simulink model "CSTR_gen_UA_err"  (R2020a)
settings: Solver=VariableStepAuto  StartTime=0.0  StopTime=dur  RelTol=1e-3
values from neighbouring files (symbols this model uses):
  Ca_i = 1    [CSTR_In.mat]
  CaSwitch = 0    [CSTR_Data_Generation.m]    (also in CSTR_Data_loops_UA_err.m)
  EaR = 8750    [CSTR_In.mat]
  H = 50000    [CSTR_In.mat]
  HA = 50000    [CSTR_In.mat]
  HD = 239    [CSTR_In.mat]
  k0Switch = 0    [CSTR_Data_Generation.m]    (also in CSTR_Data_loops_UA_err.m)
  k_0 = 72000000000    [CSTR_In.mat]
  serr = 0    [CSTR_Data_Generation.m]    (also in CSTR_Data_loops_UA_err.m)
  t_samp = 1    [CSTR_Data_Generation.m]    (also in CSTR_Data_loops_UA_err.m)
  t_Tj = 0    [CSTR_Data_Generation.m]    (also in CSTR_Data_loops_UA_err.m)
  Tj_i = 290    [CSTR_Data_Generation.m]    (also in CSTR_Data_loops_UA_err.m)
  Tj_o = Tj_i    (= 290)    [CSTR_Data_Generation.m]    (also in CSTR_Data_loops_UA_err.m)
  UASwitch = 1    [CSTR_Data_Generation.m]    (also in CSTR_Data_loops_UA_err.m)
  V = 100    [CSTR_In.mat]
libraries: simulink x7
settings Model: Creator=20029586  LastModifiedBy=20029586
settings DataIOCC: ReturnWorkspaceOutputs=off
settings DebuggingCC: ArithmeticOperatorsInVariantConditions=warning
settings SFSimCC: CustomCodeUndefinedFunction=UseInterfaceOnly
settings CodeAppCC: StateflowObjectComments=on

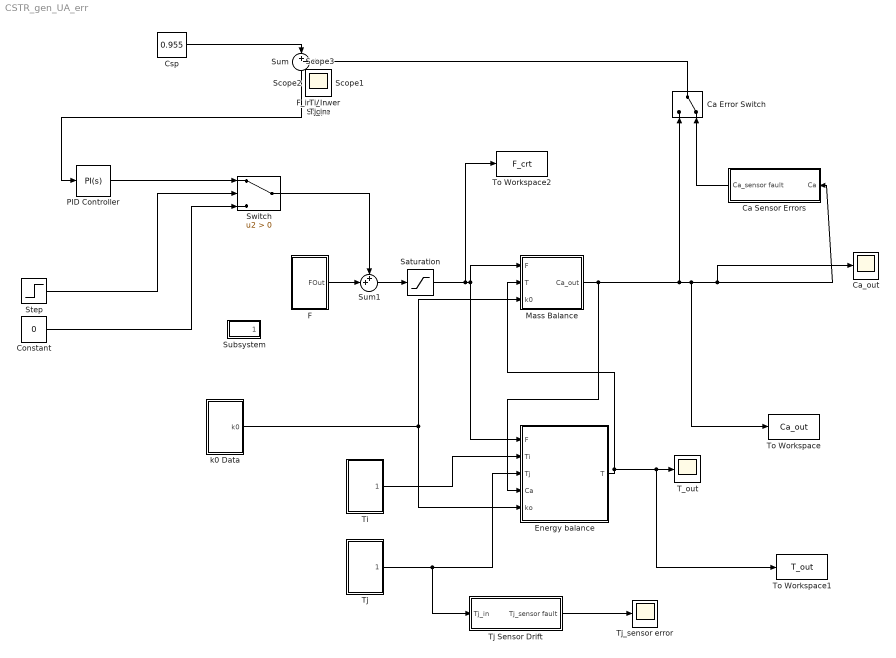
== system CSTR_gen_UA_err ==
  Ca Error Switch : ManualSwitch  CurrentSetting=0
  Ca Sensor Errors : Subsystem
  Ca_out : Scope
  Constant : Constant  Value=0
  Csp : Constant  Value=0.955
  Energy balance : Subsystem
  F : Subsystem
  Mass Balance : Subsystem
  PID Controller : simulink/Continuous/PID Controller  Controller=PI  Form=Parallel  TimeDomain=Continuous-time  UseExternalTs=off  SampleTime=-1  IntegratorMethod=Forward Euler  FilterMethod=Forward Euler  ControllerParametersSource=internal  P=5  I=50  D=0  UseFilter=on  N=100  TunerSelectOption=Transfer Function Based (PID Tuner App)  InitialConditionSource=internal  InitialConditionForIntegrator=0  InitialConditionForFilter=0  DifferentiatorICPrevScaledInput=0  ExternalReset=none  TrackingMode=off  Kt=1  LimitOutput=off  UpperSaturationLimit=inf  LowerSaturationLimit=-inf  LinearizeAsGain=on  AntiWindupMode=none  Kb=1  POutMin=[]  POutMax=[]  IOutMin=[]  IOutMax=[]  DOutMin=[]  DOutMax=[]  NOutMin=[]  NOutMax=[]  SumOutMin=[]  SumOutMax=[]  SaturationOutMin=[]  SaturationOutMax=[]  PParamMin=[]  PParamMax=[]  IParamMin=[]  IParamMax=[]  DParamMin=[]  DParamMax=[]  NParamMin=[]  NParamMax=[]  KbParamMin=[]  KbParamMax=[]  KtParamMin=[]  KtParamMax=[]  KbOutMin=[]  KbOutMax=[]  KtOutMin=[]  KtOutMax=[]  IntegratorOutMin=[]  IntegratorOutMax=[]  FilterOutMin=[]  FilterOutMax=[]  SumI1OutMin=[]  SumI1OutMax=[]  SumI2OutMin=[]  SumI2OutMax=[]  SumI3OutMin=[]  SumI3OutMax=[]  SumI4OutMin=[]  SumI4OutMax=[]  SumDOutMin=[]  SumDOutMax=[]  DifferentiatorOutMin=[]  DifferentiatorOutMax=[]  FilterDiffOutCoefMin=[]  FilterDiffOutCoefMax=[]  ReciprocalOutMin=[]  ReciprocalOutMax=[]  SumDenOutMin=[]  SumDenOutMax=[]  SumNumOutMin=[]  SumNumOutMax=[]  DivideOutMin=[]  DivideOutMax=[]  UdiffTsProdOutMin=[]  UdiffTsProdOutMax=[]  NTsProdOutMin=[]  NTsProdOutMax=[]  UintegralTsProdOutMin=[]  UintegralTsProdOutMax=[]  UngainTsProdOutMin=[]  UngainTsProdOutMax=[]  IntegratorContinuousStateAttributes=''  IntegratorStateMustResolveToSignalObject=off  IntegratorRTWStateStorageClass=Auto  FilterContinuousStateAttributes=''  FilterStateMustResolveToSignalObject=off  FilterRTWStateStorageClass=Auto  ParallelPVariant=InternalParameters  IdealPVariant=Disabled  IVariant=InternalParameters  DVariant=Disabled  IntegratorVariant=Continuous  SatVariant=Disabled  AWVariant=Passthrough  PCopyVariant=Disabled  TRVariant=Disabled  FdbkBlocksVariant=Forward  IdealPFdbkVariant=Disabled  SatFdbkVariant=Disabled  DerivativeFilterVariant=Disabled  NVariant=Disabled  NCopyVariant=Disabled_SignalSpec  FilterICVariant=Disabled  IntegratorICVariant=InternalICs  ExternalResetVariant=Disabled  TRSumVariant=Passthrough  SumFdbkVariant=Disabled  SumVariant=Sum_PI  TsampFilterVariant=InternalTs  TsampNgainVariant=Passthrough  TsampIntegralVariant=Passthrough
  Saturation : Saturate  UpperLimit=5000  LowerLimit=0
  Step : Step  Time=0  Before=-1  SampleTime=0
  Subsystem : Subsystem
  Sum : Sum  Inputs=|+-
  Sum1 : Sum  Inputs=++|
  Switch : Switch  Criteria=u2 > Threshold
  T_out : Scope
  Ti : Subsystem
  Tj : Subsystem
  Tj Sensor Drift : Subsystem
  Tj_sensor error : Scope
  To Workspace : ToWorkspace  VariableName=Ca_out  SaveFormat=Timeseries  SampleTime=t_samp
  To Workspace1 : ToWorkspace  VariableName=T_out  SaveFormat=Timeseries  SampleTime=t_samp
  To Workspace2 : ToWorkspace  VariableName=F_crt  SaveFormat=Timeseries  SampleTime=t_samp
  k0 Data : Subsystem
  F_in Viewer : Scope
  Scope{,1..3} (4 alike) : Scope
  Ti_In : Scope
  Tj_in : Scope
  wires:
  Energy balance/1(T) -> To Workspace1/1, T_out/1, Mass Balance/2(T)
  Ti/1(Ti_Out) -> Energy balance/2(Ti)
  Tj/1(Tj_Out) -> Tj Sensor Drift/1(Tj_in), Energy balance/3(Tj)
  Mass Balance/1(Ca_out) -> Ca Sensor Errors/1(Ca), Ca_out/1, To Workspace/1, Ca Error Switch/1, Energy balance/4(Ca)
  Csp/1 -> Sum/1
  F/1(FOut) -> Sum1/2
  Tj Sensor Drift/1(Tj_sensor fault) -> Tj_sensor error/1
  Ca Error Switch/1 -> Sum/2
  Ca Sensor Errors/1(Ca_sensor fault) -> Ca Error Switch/2
  Switch/1 -> Sum1/1
  Constant/1 -> Switch/3
  Step/1 -> Switch/2
  Saturation/1 -> Energy balance/1(F), Mass Balance/1(F), To Workspace2/1
  Sum1/1 -> Saturation/1
  k0 Data/1(k0) -> Mass Balance/3(k0), Energy balance/5(ko)
  PID Controller/1 -> Switch/1
  Sum/1 -> PID Controller/1

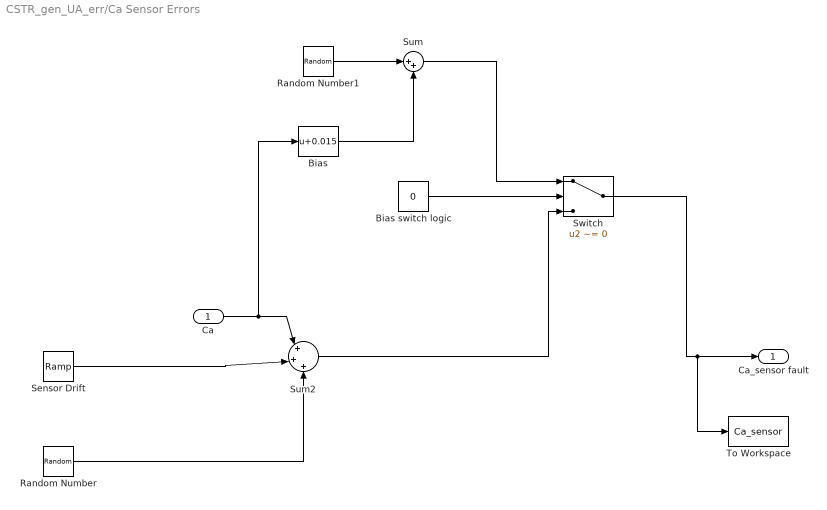
== system CSTR_gen_UA_err/Ca Sensor Errors ==
  Ca : Inport
  Bias : Bias  Bias=0.015
  Bias switch logic : Constant  Value=0
  Random Number : RandomNumber  Variance=0.0001  SampleTime=0.1
  Random Number1 : RandomNumber  Variance=1*10^-6  SampleTime=0.1
  Sensor Drift : simulink/Sources/Ramp  slope=serr  start=t_serr  InitialOutput=0
  Sum : Sum  Inputs=|++
  Sum2 : Sum  Inputs=|+|+|+
  Switch : Switch  Criteria=u2 ~= 0
  To Workspace : ToWorkspace  VariableName=Ca_sensor  SaveFormat=Timeseries  SampleTime=t_samp
  Ca_sensor fault : Outport
  wires:
  Ca/1 -> Bias/1, Sum2/1
  Sensor Drift/1 -> Sum2/2
  Sum2/1 -> Switch/3
  Random Number/1 -> Sum2/3
  Random Number1/1 -> Sum/1
  Bias/1 -> Sum/2
  Sum/1 -> Switch/1
  Bias switch logic/1 -> Switch/2
  Switch/1 -> To Workspace/1, Ca_sensor fault/1

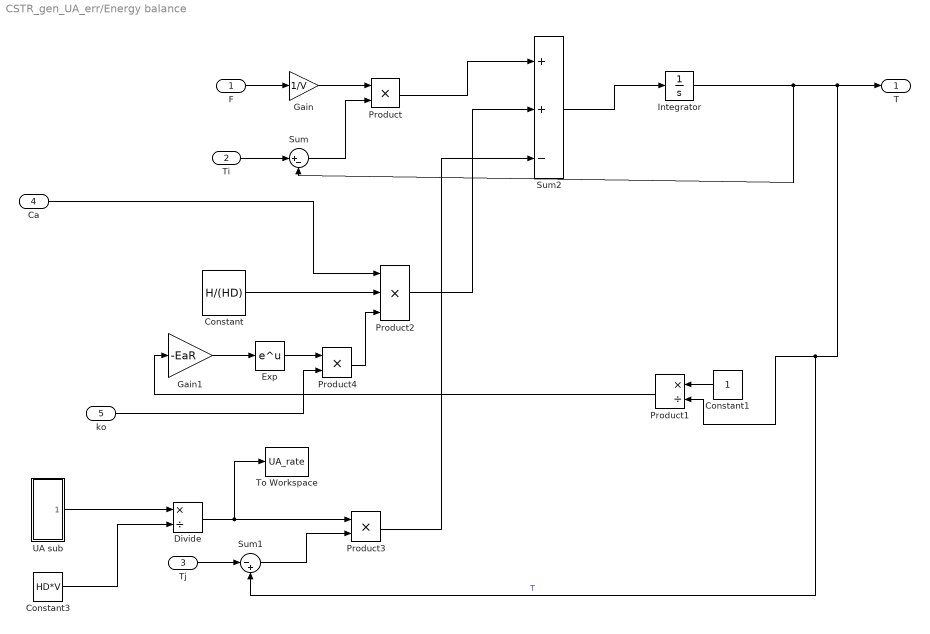
== system CSTR_gen_UA_err/Energy balance ==
  F : Inport
  Ti : Inport  Port=2
  Tj : Inport  Port=3
  Ca : Inport  Port=4
  ko : Inport  Port=5
  Constant : Constant  Value=H/(HD)
  Constant1 : Constant
  Constant3 : Constant  Value=HD*V
  Divide : Product  Inputs=*/
  Exp : Math  SignedPower=on  SaturateOnIntegerOverflow=on
  Gain : Gain  Gain=1/V
  Gain1 : Gain  Gain=-EaR
  Integrator : Integrator  InitialCondition=312.4
  Product : Product
  Product1 : Product  Inputs=*/
  Product2 : Product  Inputs=3
  Product3 : Product
  Product4 : Product
  Sum : Sum  Inputs=|+-
  Sum1 : Sum  Inputs=|-+
  Sum2 : Sum  Inputs=|++-
  To Workspace : ToWorkspace  VariableName=UA_rate  SaveFormat=Timeseries  SampleTime=t_samp
  UA sub : Subsystem
  T : Outport
  wires:
  Integrator/1 -> Sum/2, Sum1/2, Product1/2, T/1  "T"
  F/1 -> Gain/1
  Gain/1 -> Product/1
  Ti/1 -> Sum/1
  Sum/1 -> Product/2
  Constant1/1 -> Product1/1
  Product1/1 -> Gain1/1
  Gain1/1 -> Exp/1
  Exp/1 -> Product4/1
  Constant/1 -> Product2/2
  Product4/1 -> Product2/3
  Divide/1 -> To Workspace/1, Product3/1
  Tj/1 -> Sum1/1
  Sum1/1 -> Product3/2
  Product/1 -> Sum2/1
  Product2/1 -> Sum2/2
  Product3/1 -> Sum2/3
  Sum2/1 -> Integrator/1
  Ca/1 -> Product2/1
  ko/1 -> Product4/2
  Constant3/1 -> Divide/2
  UA sub/1(Out1) -> Divide/1

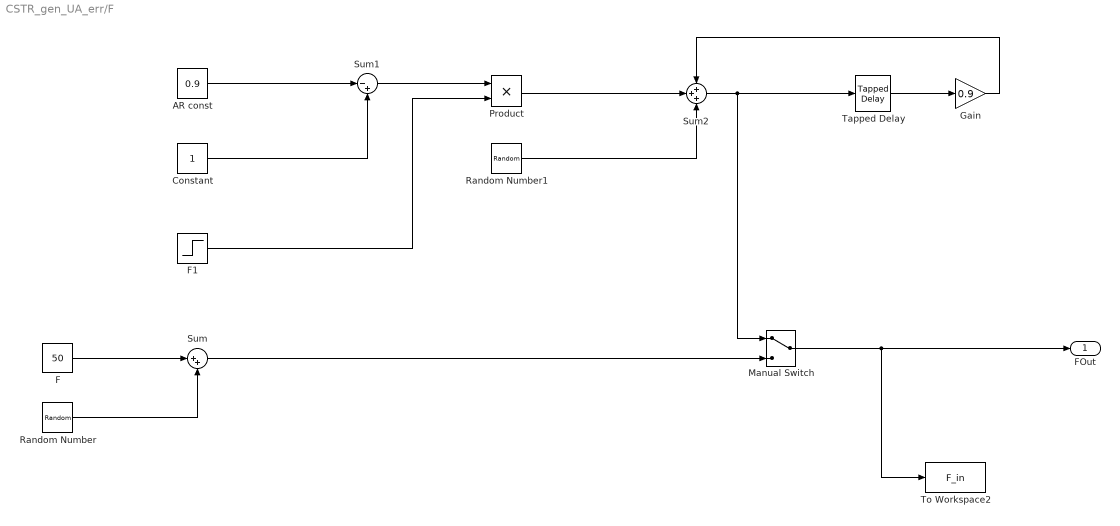
== system CSTR_gen_UA_err/F ==
  AR const : Constant  Value=0.9
  Constant : Constant
  F : Constant  Value=50
  F1 : Step  Time=0  Before=50  After=50  SampleTime=0
  Gain : Gain  Gain=0.9
  Manual Switch : ManualSwitch
  Product : Product
  Random Number : RandomNumber  Variance=1.9  SampleTime=0.1
  Random Number1 : RandomNumber  Variance=1.9  SampleTime=0.1
  Sum : Sum  Inputs=|++
  Sum1 : Sum  Inputs=|-+
  Sum2 : Sum  Inputs=+++
  Tapped Delay : simulink/Discrete/Tapped Delay  vinit=50  samptime=0.1  NumDelays=1  DelayOrder=Oldest  includeCurrent=off
  To Workspace2 : ToWorkspace  VariableName=F_in  SaveFormat=Timeseries  SampleTime=t_samp
  FOut : Outport
  wires:
  F/1 -> Sum/1
  Sum/1 -> Manual Switch/2
  Manual Switch/1 -> To Workspace2/1, FOut/1
  Random Number/1 -> Sum/2
  AR const/1 -> Sum1/1
  Constant/1 -> Sum1/2
  Sum1/1 -> Product/1
  F1/1 -> Product/2
  Product/1 -> Sum2/2
  Random Number1/1 -> Sum2/3
  Sum2/1 -> Manual Switch/1, Tapped Delay/1
  Tapped Delay/1 -> Gain/1
  Gain/1 -> Sum2/1

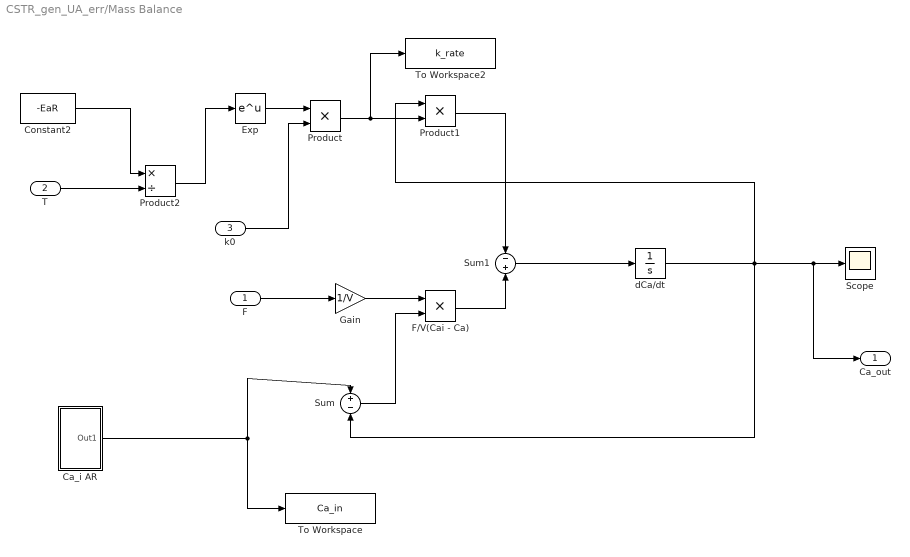
== system CSTR_gen_UA_err/Mass Balance ==
  F : Inport
  T : Inport  Port=2
  k0 : Inport  Port=3
  Ca_i AR : Subsystem
  Constant2 : Constant  Value=-EaR
  Exp : Math  SignedPower=on  SaturateOnIntegerOverflow=on
  F/V(Cai - Ca) : Product
  Gain : Gain  Gain=1/V
  Product : Product
  Product1 : Product
  Product2 : Product  Inputs=*/
  Scope : Scope
  Sum : Sum  Inputs=+-
  Sum1 : Sum  Inputs=-+
  To Workspace : ToWorkspace  VariableName=Ca_in  SaveFormat=Timeseries  SampleTime=t_samp
  To Workspace2 : ToWorkspace  VariableName=k_rate  SaveFormat=Timeseries  SampleTime=t_samp
  dCa/dt : Integrator  InitialCondition=0.952
  Ca_out : Outport
  wires:
  Product/1 -> To Workspace2/1, Product1/2
  Product1/1 -> Sum1/1
  Sum/1 -> F/V(Cai - Ca)/2
  dCa/dt/1 -> Ca_out/1, Scope/1, Sum/2, Product1/1
  Gain/1 -> F/V(Cai - Ca)/1
  Sum1/1 -> dCa/dt/1
  F/1 -> Gain/1
  Exp/1 -> Product/1
  F/V(Cai - Ca)/1 -> Sum1/2
  Constant2/1 -> Product2/1
  Product2/1 -> Exp/1
  T/1 -> Product2/2
  Ca_i AR/1(Out1) -> Sum/1, To Workspace/1
  k0/1 -> Product/2

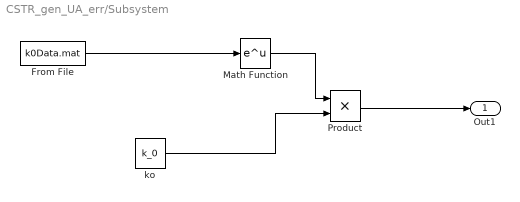
== system CSTR_gen_UA_err/Subsystem ==
  From File : FromFile  FileName=k0Data.mat  SampleTime=0.01
  Math Function : Math  SignedPower=on  SaturateOnIntegerOverflow=on
  Product : Product
  ko : Constant  Value=k_0
  Out1 : Outport
  wires:
  Math Function/1 -> Product/1
  Product/1 -> Out1/1
  From File/1 -> Math Function/1
  ko/1 -> Product/2

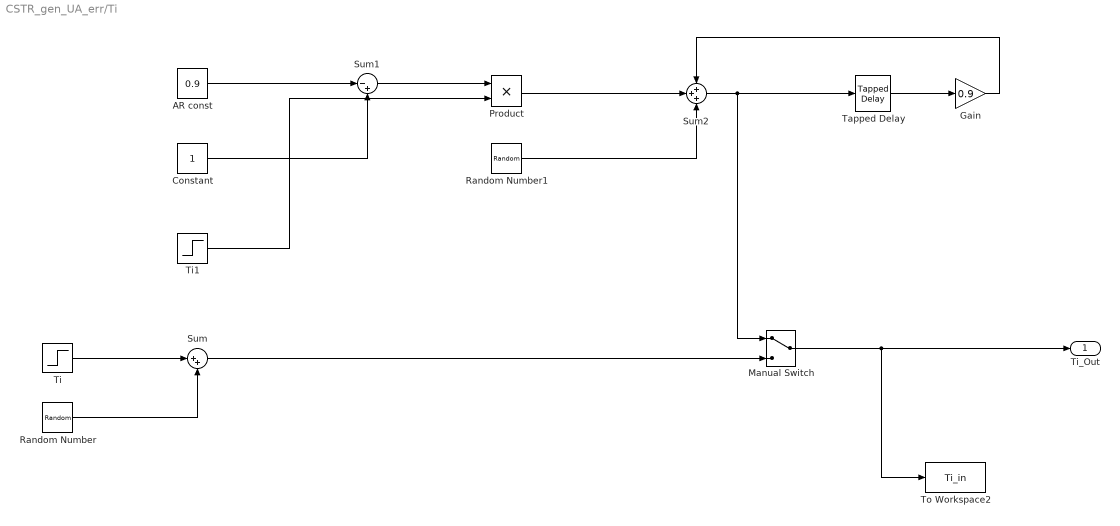
== system CSTR_gen_UA_err/Ti ==
  AR const : Constant  Value=0.9
  Constant : Constant
  Gain : Gain  Gain=0.9
  Manual Switch : ManualSwitch
  Product : Product
  Random Number : RandomNumber  Variance=0.475  SampleTime=0.1
  Random Number1 : RandomNumber  Variance=0.475  SampleTime=0.1
  Sum : Sum  Inputs=|++
  Sum1 : Sum  Inputs=|-+
  Sum2 : Sum  Inputs=+++
  Tapped Delay : simulink/Discrete/Tapped Delay  vinit=350  samptime=0.1  NumDelays=1  DelayOrder=Oldest  includeCurrent=off
  Ti : Step  Time=0  Before=350  After=350  SampleTime=0
  Ti1 : Step  Time=0  Before=350  After=350  SampleTime=0
  To Workspace2 : ToWorkspace  VariableName=Ti_in  SaveFormat=Timeseries  SampleTime=t_samp
  Ti_Out : Outport
  wires:
  Ti/1 -> Sum/1
  Sum/1 -> Manual Switch/2
  Manual Switch/1 -> To Workspace2/1, Ti_Out/1
  Random Number/1 -> Sum/2
  AR const/1 -> Sum1/1
  Constant/1 -> Sum1/2
  Sum1/1 -> Product/1
  Ti1/1 -> Product/2
  Product/1 -> Sum2/2
  Random Number1/1 -> Sum2/3
  Sum2/1 -> Manual Switch/1, Tapped Delay/1
  Tapped Delay/1 -> Gain/1
  Gain/1 -> Sum2/1

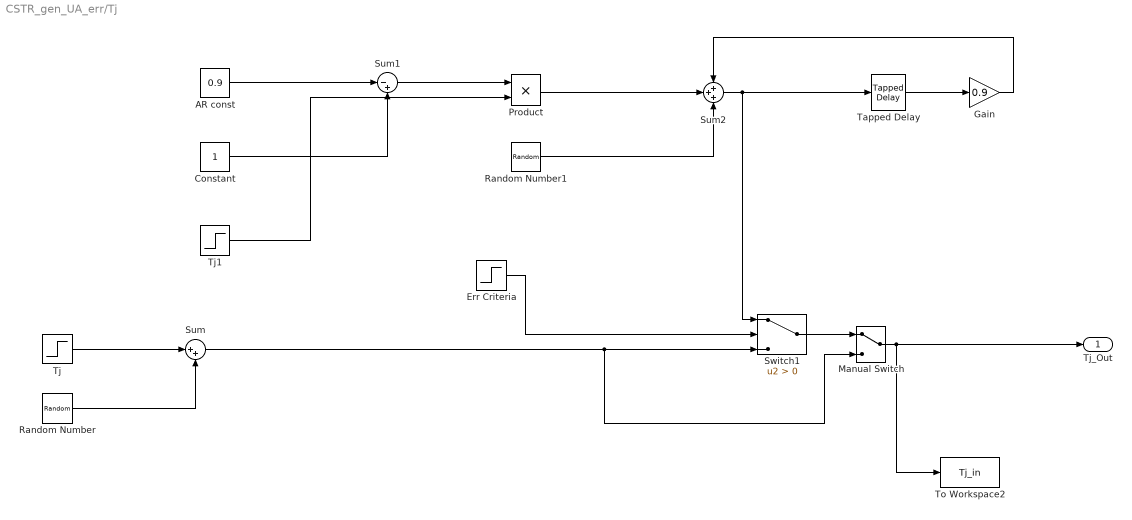
== system CSTR_gen_UA_err/Tj ==
  AR const : Constant  Value=0.9
  Constant : Constant
  Err Criteria : Step  Time=0  SampleTime=0
  Gain : Gain  Gain=0.9
  Manual Switch : ManualSwitch
  Product : Product
  Random Number : RandomNumber  Variance=0.005  SampleTime=0.1
  Random Number1 : RandomNumber  Variance=0.005  SampleTime=0.1
  Sum : Sum  Inputs=|++
  Sum1 : Sum  Inputs=|-+
  Sum2 : Sum  Inputs=+++
  Switch1 : Switch  Criteria=u2 > Threshold
  Tapped Delay : simulink/Discrete/Tapped Delay  vinit=290  samptime=-1  NumDelays=1  DelayOrder=Oldest  includeCurrent=off
  Tj : Step  Time=10  Before=290  After=290  SampleTime=0
  Tj1 : Step  Time=t_Tj  Before=Tj_i  After=Tj_o  SampleTime=0
  To Workspace2 : ToWorkspace  VariableName=Tj_in  SaveFormat=Timeseries  SampleTime=0.1
  Tj_Out : Outport
  wires:
  Tj/1 -> Sum/1
  Sum/1 -> Manual Switch/2, Switch1/3
  Manual Switch/1 -> To Workspace2/1, Tj_Out/1
  Random Number/1 -> Sum/2
  AR const/1 -> Sum1/1
  Constant/1 -> Sum1/2
  Sum1/1 -> Product/1
  Tj1/1 -> Product/2
  Product/1 -> Sum2/2
  Random Number1/1 -> Sum2/3
  Sum2/1 -> Switch1/1, Tapped Delay/1
  Tapped Delay/1 -> Gain/1
  Gain/1 -> Sum2/1
  Err Criteria/1 -> Switch1/2
  Switch1/1 -> Manual Switch/1

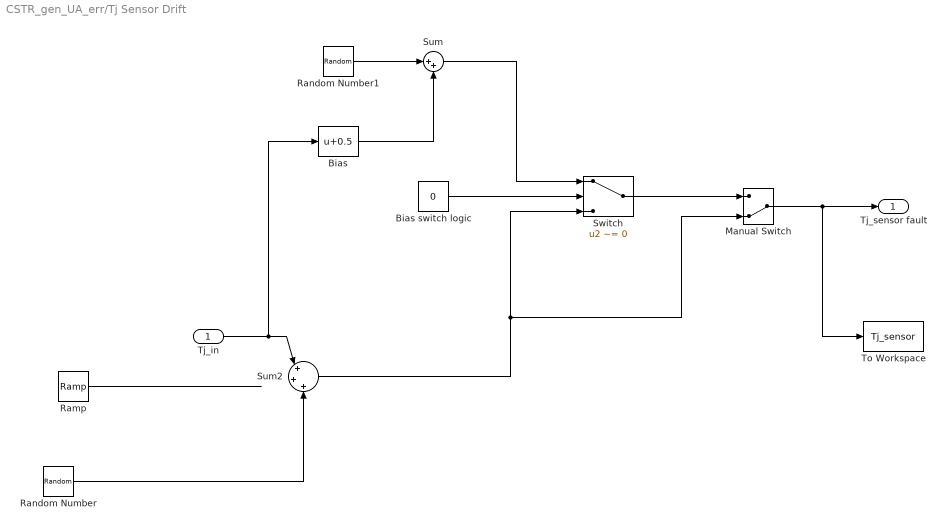
== system CSTR_gen_UA_err/Tj Sensor Drift ==
  Tj_in : Inport
  Bias : Bias  Bias=0.5
  Bias switch logic : Constant  Value=0
  Manual Switch : ManualSwitch  CurrentSetting=0
  Ramp : simulink/Sources/Ramp  slope=0.1  start=30  InitialOutput=0
  Random Number : RandomNumber  Variance=0.05  SampleTime=0.1
  Random Number1 : RandomNumber  Variance=0.05  SampleTime=0.1
  Sum : Sum  Inputs=|++
  Sum2 : Sum  Inputs=|+|+|+
  Switch : Switch  Criteria=u2 ~= 0
  To Workspace : ToWorkspace  VariableName=Tj_sensor  SaveFormat=Timeseries  SampleTime=t_samp
  Tj_sensor fault : Outport
  wires:
  Ramp/1 -> ?
  Random Number/1 -> Sum2/3
  Tj_in/1 -> Bias/1, Sum2/1
  Sum/1 -> Switch/1
  Bias switch logic/1 -> Switch/2
  Sum2/1 -> Manual Switch/2, Switch/3
  Random Number1/1 -> Sum/1
  Bias/1 -> Sum/2
  Switch/1 -> Manual Switch/1
  Manual Switch/1 -> To Workspace/1, Tj_sensor fault/1

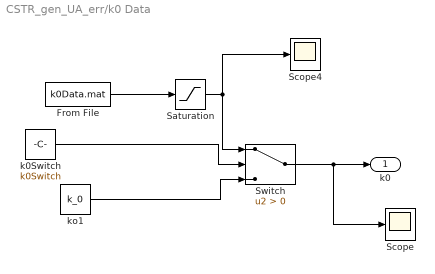
== system CSTR_gen_UA_err/k0 Data ==
  From File : FromFile  FileName=k0Data.mat  SampleTime=0.01
  Saturation : Saturate  UpperLimit=10e10  LowerLimit=0
  Scope : Scope
  Scope4 : Scope
  Switch : Switch  Criteria=u2 > Threshold
  k0Switch : Constant  Value=k0Switch
  ko1 : Constant  Value=k_0
  k0 : Outport
  wires:
  From File/1 -> Saturation/1
  Switch/1 -> Scope/1, k0/1
  ko1/1 -> Switch/3
  k0Switch/1 -> Switch/2
  Saturation/1 -> Switch/1, Scope4/1

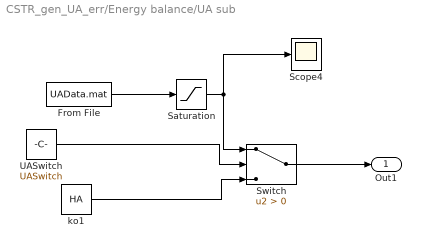
== system CSTR_gen_UA_err/Energy balance/UA sub ==
  From File : FromFile  FileName=UAData.mat  SampleTime=0.01
  Saturation : Saturate  UpperLimit=60000  LowerLimit=0
  Scope4 : Scope
  Switch : Switch  Criteria=u2 > Threshold
  UASwitch : Constant  Value=UASwitch
  ko1 : Constant  Value=HA
  Out1 : Outport
  wires:
  Saturation/1 -> Switch/1, Scope4/1
  UASwitch/1 -> Switch/2
  From File/1 -> Saturation/1
  Switch/1 -> Out1/1
  ko1/1 -> Switch/3

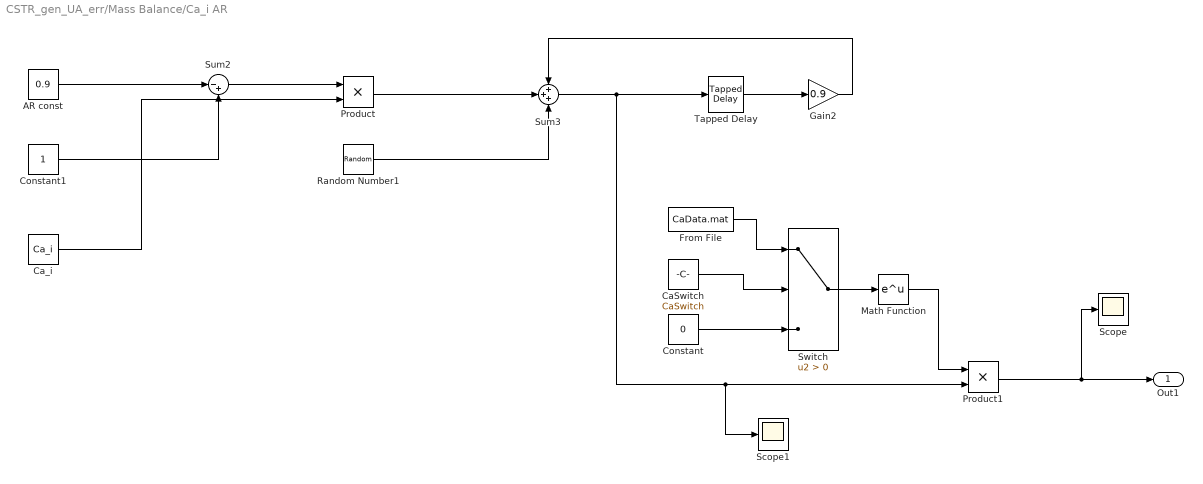
== system CSTR_gen_UA_err/Mass Balance/Ca_i AR ==
  AR const : Constant  Value=0.9
  CaSwitch : Constant  Value=CaSwitch
  Ca_i : Constant  Value=Ca_i
  Constant : Constant  Value=0
  Constant1 : Constant
  From File : FromFile  FileName=CaData.mat  SampleTime=0.01
  Gain2 : Gain  Gain=0.9
  Math Function : Math  SignedPower=on  SaturateOnIntegerOverflow=on
  Product : Product
  Product1 : Product
  Random Number1 : RandomNumber  Variance=0.00002  SampleTime=0.1
  Scope : Scope
  Scope1 : Scope
  Sum2 : Sum  Inputs=|-+
  Sum3 : Sum  Inputs=+++
  Switch : Switch  Criteria=u2 > Threshold
  Tapped Delay : simulink/Discrete/Tapped Delay  vinit=Ca_i  samptime=0.1  NumDelays=1  DelayOrder=Oldest  includeCurrent=off
  Out1 : Outport
  wires:
  Ca_i/1 -> Product/2
  Sum2/1 -> Product/1
  AR const/1 -> Sum2/1
  Product/1 -> Sum3/2
  Tapped Delay/1 -> Gain2/1
  Constant1/1 -> Sum2/2
  Random Number1/1 -> Sum3/3
  Gain2/1 -> Sum3/1
  From File/1 -> Switch/1
  Product1/1 -> Scope/1, Out1/1
  Sum3/1 -> Scope1/1, Product1/2, Tapped Delay/1
  Math Function/1 -> Product1/1
  Switch/1 -> Math Function/1
  CaSwitch/1 -> Switch/2
  Constant/1 -> Switch/3
